simulink model "practice"  (R2018a)
settings: Solver=VariableStepAuto  StartTime=0.0  StopTime=10.0  RelTol=1e-3
settings Model: Creator=Liuinuy  LastModifiedBy=Liuinuy

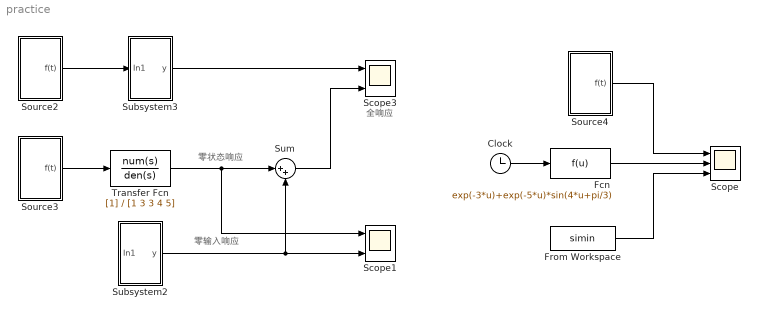
== system practice ==
  note: 零状态响应
  note: 全响应
  note: 零输入响应
  Clock : Clock
  Fcn : Fcn  Expr=exp(-3*u)+exp(-5*u)*sin(4*u+pi/3)
  From Workspace : FromWorkspace  VariableName=simin  SampleTime=0.1
  Scope : Scope  NumInputPorts=3
  Scope1 : Scope  NumInputPorts=2
  Scope3 : Scope  NumInputPorts=2
  Source2 : Subsystem  mask{amp=1, w=4, phase=pi/3, D1=-3, D2=-5}
      mask prompts: amp "Amplitude"; w "Frequency"
      mask DialogControl Control2 Prompt: nothing
  Source3 : Subsystem  mask{amp=1, w=4, phase=pi/3, D1=-3, D2=-5}
      mask prompts: amp "Amplitude"; w "Frequency"
      mask DialogControl Control2 Prompt: nothing
  Source4 : Subsystem  mask{amp=1, w=4, phase=pi/3, D1=-3, D2=-5}
      mask prompts: amp "Amplitude"; w "Frequency"
      mask DialogControl Control2 Prompt: nothing
  Subsystem2 : Subsystem  mask(f1){y3=0.2, y2=0.5, y1=0.5, y0=1, c1=3, c2=3, c3=4, c4=5}
      mask prompts: y3 "y'''(0)"; y2 "y''(0)"; y1 "y'(0)"; y0 "y(0)"
  Subsystem3 : Subsystem  mask(f1){y3=0.2, y2=0.5, y1=0.5, y0=1, c1=3, c2=3, c3=4, c4=5}
      mask prompts: y3 "y'''(0)"; y2 "y''(0)"; y1 "y'(0)"; y0 "y(0)"
  Sum : Sum  Inputs=|++
  Transfer Fcn : TransferFcn  Denominator=[1 3 3 4 5]
  wires:
  Source2/1(f(t)) -> Subsystem3/1(In1)
  Subsystem3/1(y) -> Scope3/1
  Source3/1(f(t)) -> Transfer Fcn/1
  Clock/1 -> Fcn/1
  Fcn/1 -> Scope/2
  From Workspace/1 -> Scope/3
  Source4/1(f(t)) -> Scope/1
  Subsystem2/1(y) -> Scope1/2, Sum/2
  Transfer Fcn/1 -> Scope1/1, Sum/1
  Sum/1 -> Scope3/2

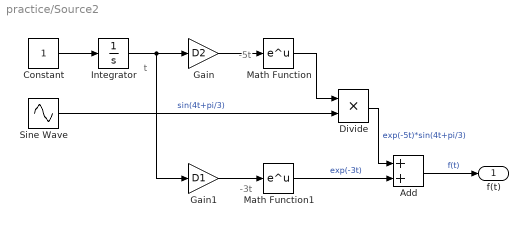
== system practice/Source2 ==
  note: t
  note: -5t
  note: -3t
  Add : Sum
  Constant : Constant
  Divide : Product  Inputs=**
  Gain : Gain  Gain=D2
  Gain1 : Gain  Gain=D1
  Integrator : Integrator
  Math Function : Math  SaturateOnIntegerOverflow=on
  Math Function1 : Math  SaturateOnIntegerOverflow=on
  Sine Wave : Sin  Amplitude=amp  Frequency=w  Phase=phase  SampleTime=0
  f(t) : Outport
  wires:
  Sine Wave/1 -> Divide/2  "sin(4t+pi/3)"
  Constant/1 -> Integrator/1
  Divide/1 -> Add/1  "exp(-5t)*sin(4t+pi/3)"
  Math Function1/1 -> Add/2  "exp(-3t)"
  Math Function/1 -> Divide/1
  Add/1 -> f(t)/1  "f(t)"
  Gain1/1 -> Math Function1/1
  Integrator/1 -> Gain/1, Gain1/1
  Gain/1 -> Math Function/1

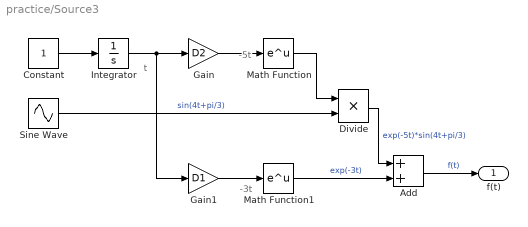
== system practice/Source3 ==
  note: t
  note: -5t
  note: -3t
  Add : Sum
  Constant : Constant
  Divide : Product  Inputs=**
  Gain : Gain  Gain=D2
  Gain1 : Gain  Gain=D1
  Integrator : Integrator
  Math Function : Math  SaturateOnIntegerOverflow=on
  Math Function1 : Math  SaturateOnIntegerOverflow=on
  Sine Wave : Sin  Amplitude=amp  Frequency=w  Phase=phase  SampleTime=0
  f(t) : Outport
  wires:
  Sine Wave/1 -> Divide/2  "sin(4t+pi/3)"
  Constant/1 -> Integrator/1
  Divide/1 -> Add/1  "exp(-5t)*sin(4t+pi/3)"
  Math Function1/1 -> Add/2  "exp(-3t)"
  Math Function/1 -> Divide/1
  Add/1 -> f(t)/1  "f(t)"
  Gain1/1 -> Math Function1/1
  Integrator/1 -> Gain/1, Gain1/1
  Gain/1 -> Math Function/1

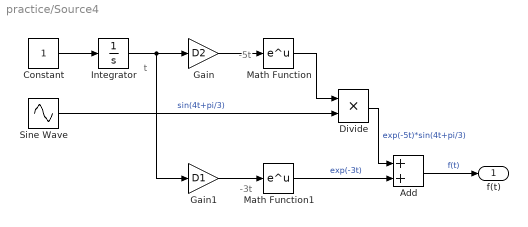
== system practice/Source4 ==
  note: t
  note: -5t
  note: -3t
  Add : Sum
  Constant : Constant
  Divide : Product  Inputs=**
  Gain : Gain  Gain=D2
  Gain1 : Gain  Gain=D1
  Integrator : Integrator
  Math Function : Math  SaturateOnIntegerOverflow=on
  Math Function1 : Math  SaturateOnIntegerOverflow=on
  Sine Wave : Sin  Amplitude=amp  Frequency=w  Phase=phase  SampleTime=0
  f(t) : Outport
  wires:
  Sine Wave/1 -> Divide/2  "sin(4t+pi/3)"
  Constant/1 -> Integrator/1
  Divide/1 -> Add/1  "exp(-5t)*sin(4t+pi/3)"
  Math Function1/1 -> Add/2  "exp(-3t)"
  Math Function/1 -> Divide/1
  Add/1 -> f(t)/1  "f(t)"
  Gain1/1 -> Math Function1/1
  Integrator/1 -> Gain/1, Gain1/1
  Gain/1 -> Math Function/1

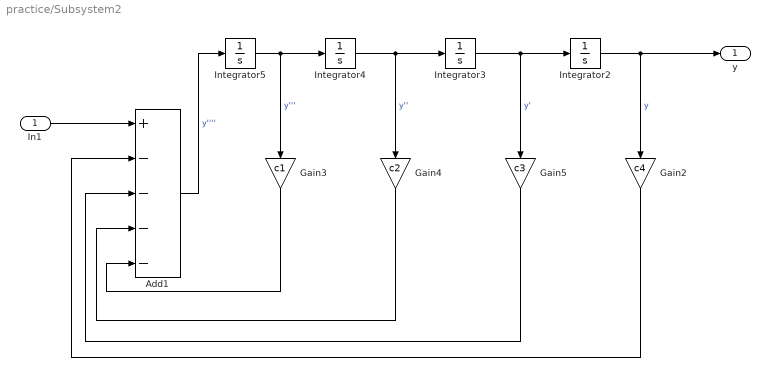
== system practice/Subsystem2 ==
  In1 : Inport
  Add1 : Sum  Inputs=+----
  Gain2 : Gain  Gain=c4
  Gain3 : Gain  Gain=c1
  Gain4 : Gain  Gain=c2
  Gain5 : Gain  Gain=c3
  Integrator2 : Integrator  InitialCondition=y0
  Integrator3 : Integrator  InitialCondition=y1
  Integrator4 : Integrator  InitialCondition=y2
  Integrator5 : Integrator  InitialCondition=y3
  y : Outport
  wires:
  Gain4/1 -> Add1/4
  Add1/1 -> Integrator5/1  "y''''"
  Gain3/1 -> Add1/5
  Integrator5/1 -> Gain3/1, Integrator4/1  "y'''"
  Integrator4/1 -> Gain4/1, Integrator3/1  "y''"
  In1/1 -> Add1/1
  Integrator2/1 -> Gain2/1, y/1  "y"
  Gain5/1 -> Add1/3
  Gain2/1 -> Add1/2
  Integrator3/1 -> Gain5/1, Integrator2/1  "y'"

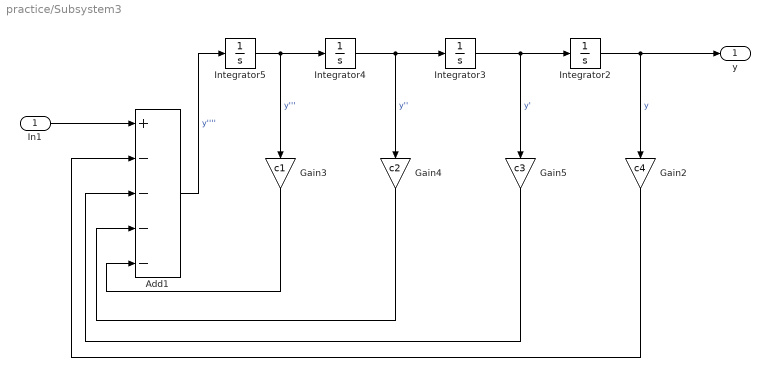
== system practice/Subsystem3 ==
  In1 : Inport
  Add1 : Sum  Inputs=+----
  Gain2 : Gain  Gain=c4
  Gain3 : Gain  Gain=c1
  Gain4 : Gain  Gain=c2
  Gain5 : Gain  Gain=c3
  Integrator2 : Integrator  InitialCondition=y0
  Integrator3 : Integrator  InitialCondition=y1
  Integrator4 : Integrator  InitialCondition=y2
  Integrator5 : Integrator  InitialCondition=y3
  y : Outport
  wires:
  Integrator3/1 -> Integrator2/1, Gain5/1  "y'"
  Gain2/1 -> Add1/2
  Gain5/1 -> Add1/3
  Integrator2/1 -> y/1, Gain2/1  "y"
  In1/1 -> Add1/1
  Integrator4/1 -> Integrator3/1, Gain4/1  "y''"
  Integrator5/1 -> Integrator4/1, Gain3/1  "y'''"
  Gain3/1 -> Add1/5
  Add1/1 -> Integrator5/1  "y''''"
  Gain4/1 -> Add1/4
